simulink model "model"  (R2022a)
settings: Solver=FixedStepAuto  StartTime=0.0  StopTime=10.0  RelTol=1e-3  EnableMultiTasking=on
libraries: arduinolib x1
settings Model: ExtModeTrigDuration=2  Creator=kojirotanakamba  LastModifiedBy=kojirotanakamba
settings OptimizationCC: DefaultParameterBehavior=Inlined  EnhancedBackFolding=on  PassReuseOutputArgsAs=Individual arguments  ZeroExternalMemoryAtStartup=off  ZeroInternalMemoryAtStartup=off  MaxStackSize=64  OptimizeBlockOrder=speed  DifferentSizesBufferReuse=on  OptimizationCustomize=off  EfficientTunableParamExpr=on
settings DebuggingCC: ParameterTunabilityLossMsg=error
settings HardwareCC: ProdBitPerPointer=32  ProdBitPerSizeT=32  ProdBitPerPtrDiffT=32  ProdLargestAtomicInteger=Long  ProdLargestAtomicFloat=Double  ProdWordSize=32  ProdHWDeviceType=ARM Compatible->ARM Cortex
settings SFSimCC: MATLABDynamicMemAlloc=off
settings RTWCC: SystemTargetFile=ert.tlc  HardwareBoard=Arduino Due  GenCodeOnly=on  TemplateMakefile=ert_default_tmf  Toolchain=Arduino ARM  BuildConfiguration=Faster Runs
settings CodeAppCC: ForceParamTrailComments=on  IgnoreCustomStorageClasses=off  OperatorAnnotations=on  SimulinkDataObjDesc=on  SFDataObjDesc=on  InsertBlockDesc=on
settings ERTTargetCC: TargetLangStandard=C99 (ISO)  InlinedParameterPlacement=NonHierarchical  ERTCustomFileTemplate=example_file_process.tlc

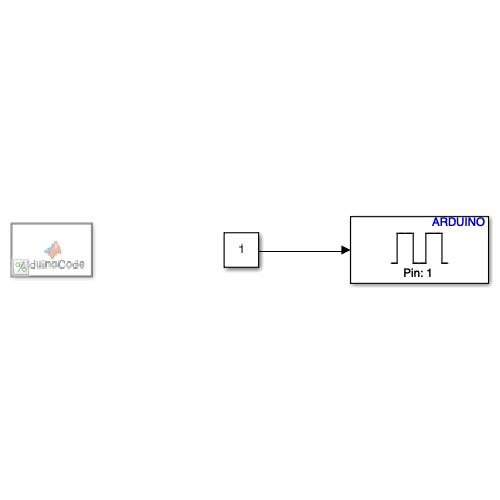
[thumbnail: Simulink's stored preview of the top-level diagram]
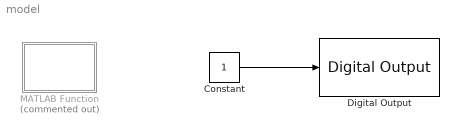
== system model ==
  Constant : Constant
  Digital Output : arduinolib/Digital Output  pinNumber=1  Direction=output  blockPlatform=arduino
  MATLAB Function : MATLAB Function  Commented=on  TreatAsAtomicUnit=on
  wires:
  Constant/1 -> Digital Output/1

== matlab function model/MATLAB Function ==
function arduinoCode

    persistent arduinoObj

    if(isempty(arduinoObj))
        arduinoObj = arduino();
        configurePin(arduinoObj, 'D1', 'DigitalOutput');
        configurePin(arduinoObj, 'D2', 'DigitalInput');
    end

    writeDigitalPin(arduinoObj, 'D1', 1);
    readDigitalPin(arduinoObj, 'D2');
